simulink model "CartPendulum_sim"  (R2016a)
settings: Solver=ode45  StartTime=0.0  StopTime=15  RelTol=1e-4
libraries: cstblocks x6
settings Model: Creator=fbianchi  LastModifiedBy=ferna
settings DataIOCC: LimitDataPoints=on  SaveFormat=Array
settings DebuggingCC: UnderspecifiedInitializationDetection=Classic  MergeDetectMultiDrivingBlocksExec=none  SolverPrmCheckMsg=warning  StateNameClashWarn=warning
settings HardwareCC: ProdBitPerPointer=32  ProdLargestAtomicFloat=None  ProdIntDivRoundTo=Undefined  ProdEndianess=Unspecified  ProdWordSize=32  ProdHWDeviceType=32-bit Generic
settings ModelReferenceCC: PropagateSignalLabelsOutOfModel=off
settings ConfigComp: CovModelRefEnable=Off

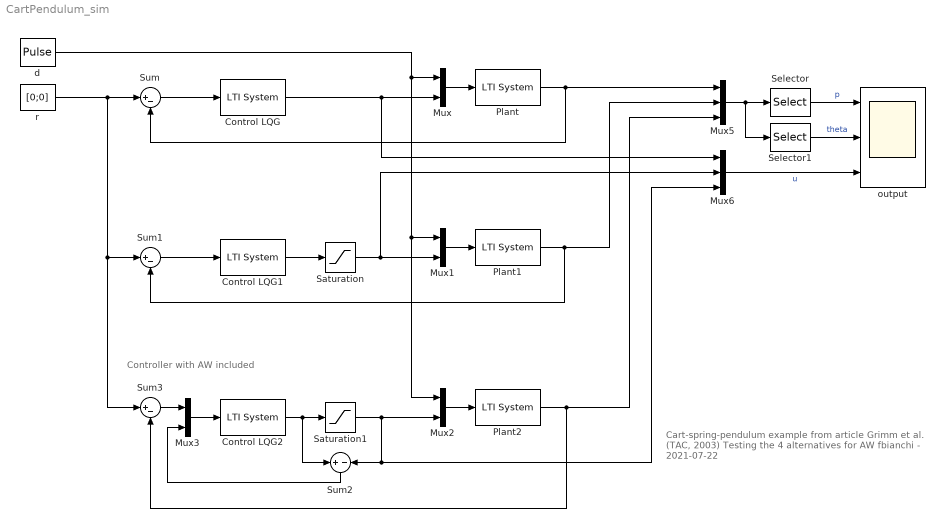
== system CartPendulum_sim ==
  note: Controller with AW included
  note: Cart-spring-pendulum example from article
      | Grimm et al. (TAC, 2003)
      |
      | Testing the 4 alternatives for AW
      |
      | fbianchi - 2021-07-22
  Control LQG : cstblocks/LTI System  sys=Klqg  IC=[]
  Control LQG1 : cstblocks/LTI System  sys=Klqg  IC=[]
  Control LQG2 : cstblocks/LTI System  sys=Kaw  IC=[]
  Mux : Mux  Inputs=2
  Mux1 : Mux  Inputs=2
  Mux2 : Mux  Inputs=2
  Mux3 : Mux  Inputs=[2 1]
  Mux5 : Mux  Inputs=[2 2 2]
  Mux6 : Mux  Inputs=3
  Plant : cstblocks/LTI System  sys=G  IC=[]
  Plant1 : cstblocks/LTI System  sys=G  IC=[]
  Plant2 : cstblocks/LTI System  sys=G  IC=[]
  Saturation : Saturate  UpperLimit=5  LowerLimit=-5
  Saturation1 : Saturate  UpperLimit=5  LowerLimit=-5
  Selector : Selector  InputPortWidth=6  IndexOptions=Index vector (dialog)  Indices=[1 3 5]  OutputSizes=1
  Selector1 : Selector  InputPortWidth=6  IndexOptions=Index vector (dialog)  Indices=[2 4 6]  OutputSizes=1
  Sum : Sum  Inputs=|+-
  Sum1 : Sum  Inputs=|+-
  Sum2 : Sum  Inputs=+-
  Sum3 : Sum  Inputs=|+-
  d : DiscretePulseGenerator  PulseType=Time based  Amplitude=1.6  Period=100  PulseWidth=0.05  PhaseDelay=1
  output : Scope  NumInputPorts=3
  r : Constant  Value=[0;0]
  wires:
  Control LQG/1 -> Mux6/1, Mux/2
  Mux/1 -> Plant/1
  Sum/1 -> Control LQG/1
  Plant/1 -> Sum/2, Mux5/1
  Control LQG1/1 -> Saturation/1
  Mux1/1 -> Plant1/1
  Sum1/1 -> Control LQG1/1
  Plant1/1 -> Mux5/2, Sum1/2
  Saturation/1 -> Mux6/2, Mux1/2
  d/1 -> Mux2/1, Mux1/1, Mux/1
  Control LQG2/1 -> Sum2/1, Saturation1/1
  Mux2/1 -> Plant2/1
  Saturation1/1 -> Mux6/3, Sum2/2, Mux2/2
  Mux3/1 -> Control LQG2/1
  r/1 -> Sum3/1, Sum1/1, Sum/1
  Sum3/1 -> Mux3/1
  Plant2/1 -> Sum3/2, Mux5/3
  Mux5/1 -> Selector1/1, Selector/1
  Selector/1 -> output/1  "p"
  Mux6/1 -> output/3  "u"
  Selector1/1 -> output/2  "theta"
  Sum2/1 -> Mux3/2
